simulink library "HDL_ieee_8021513"  (R2024a)
settings: Solver=FixedStepDiscrete  StartTime=0.0  StopTime=10.0  RelTol=1e-3
undefined symbols (not defined in the file or in its folder): Add, axiWidth, channelCyclicPrefixLen, channelDataCarriers, channelEstReference, channelLUT, channelOFDMSamples, channelScramblerInit, decimatorDelay, decimatorFilter, fPHY, frequencyOffsetTimeWindow, fs, headerBitsPerFec, headerBitsPerOFDMSymbol, headerBitsPerSubcarrier, headerCyclicPrefixLen, headerDataCarriers, headerOFDMSamples, headerScramblerInit, interpolatorDelay, interpolatorFilter, leftGuard, N, ncoCarrierFrequency, ncoWordLength, numDataCarriers, oversamplingFactor, payloadBitsPerFec, payloadScramblerInit, payloadWordsPerBlock0, peakDetectorThreshold, peakDetectorWindow, preambleCyclicPrefixLen, preambleDataCarriers, preambleLUT, preambleOFDMSamples, preambleScramblerInit, QAM, rightGuard, Shift
libraries: hdlsllib x198, $bdroot x80, whdlutilities x28, whdledac x10, whdlmod x7, simulink x4, dsphdlfiltering2 x2, dsphdlsigops2 x2, commhdlcrc x2, dspsigops x2, dspstat3 x2, commdigbbndam3 x2
(part 3 of 5)

== system HDL_ieee_8021513/qam_mod ==
  data_in : Inport
  valid_in : Inport  Port=2
  bits_per_subcarrier : Inport  Port=3
  BPSK Modulator Baseband : commdigbbndpm3/BPSK Modulator Baseband  Ph=0  outDtype=Fixed-point  outWordLen=16  outUDDataType=sfix(16)  outFracLenMode=User-defined  outFracLen=14  outDataTypeStr=fixdt(1,16,14)  outLastDataTypeStr=fixdt(1,16,14)
      settings: LibrarySourceBlock=|
      | commhdldigbbndpm/BPSK
      | Modulator
      | Baseband
  Bit Slice : hdlsllib/Logic and Bit Operations/Bit Slice  lidx=0  ridx=0
  Bit Slice1 : hdlsllib/Logic and Bit Operations/Bit Slice  lidx=1  ridx=0
  Bit Slice2 : hdlsllib/Logic and Bit Operations/Bit Slice  lidx=3  ridx=0
  Constant{1..10} (10 alike) : Constant  Value=0  OutDataTypeStr=Inherit: Inherit via back propagation  SampleTime=-1  LockScale=on
  Delay : Delay  DelayLength=1  InitialCondition=0  UseCircularBuffer=on
  Delay1 : Delay  DelayLength=1  InitialCondition=0  UseCircularBuffer=on
  Multiport Switch : MultiPortSwitch  DataPortOrder=Zero-based contiguous  Inputs=8  zeroidx=on  SaturateOnIntegerOverflow=off
  Real-Imag to Complex{1..5} (5 alike) : RealImagToComplex
  batID 1 : commdigbbndam3/Rectangular QAM Modulator Baseband  M=4  InType=Integer  Enc=User-defined  Mapping=qamTwoBits  PowType=Average Power  MinDist=2  AvgPow=1  PeakPow=1  Ph=0  outDtype=Fixed-point  outWordLen=16  outUDDataType=sfix(16)  outFracLenMode=User-defined  outFracLen=14  outDataTypeStr=fixdt(1,16,14)  outLastDataTypeStr=fixdt(1,16,14)
      settings: LibrarySourceBlock=|
      | commhdldigbbndam/Rectangular QAM
      | Modulator
      | Baseband
  batID 8 : commdigbbndam3/Rectangular QAM Modulator Baseband  M=16  InType=Integer  Enc=User-defined  Mapping=qamFourBits  PowType=Average Power  MinDist=2  AvgPow=1  PeakPow=1  Ph=0  outDtype=Fixed-point  outWordLen=16  outUDDataType=sfix(16)  outFracLenMode=User-defined  outFracLen=14  outDataTypeStr=fixdt(1,16,14)  outLastDataTypeStr=fixdt(1,16,14)
      settings: LibrarySourceBlock=|
      | commhdldigbbndam/Rectangular QAM
      | Modulator
      | Baseband
  data_out : Outport
  valid_out : Outport  Port=2  VectorParamsAs1DForOutWhenUnconnected=off
  wires:
  Real-Imag to Complex5/1 -> Multiport Switch/8
  Constant10/1 -> Real-Imag to Complex5/2
  Constant9/1 -> Real-Imag to Complex5/1
  Constant1/1 -> Real-Imag to Complex4/1
  Constant8/1 -> Real-Imag to Complex4/2
  Constant6/1 -> Real-Imag to Complex3/1
  Constant7/1 -> Real-Imag to Complex3/2
  Constant2/1 -> Real-Imag to Complex2/1
  Constant4/1 -> Real-Imag to Complex2/2
  Constant5/1 -> Real-Imag to Complex1/2
  Real-Imag to Complex1/1 -> Multiport Switch/2
  Constant3/1 -> Real-Imag to Complex1/1
  BPSK Modulator Baseband/1 -> Multiport Switch/3
  Delay/1 -> data_out/1
  Real-Imag to Complex2/1 -> Multiport Switch/5
  Real-Imag to Complex4/1 -> Multiport Switch/9
  Real-Imag to Complex3/1 -> Multiport Switch/7
  batID 8/1 -> Multiport Switch/6
  batID 1/1 -> Multiport Switch/4
  Bit Slice2/1 -> batID 8/1
  Bit Slice1/1 -> batID 1/1
  Bit Slice/1 -> BPSK Modulator Baseband/1
  Multiport Switch/1 -> Delay/1
  bits_per_subcarrier/1 -> Multiport Switch/1
  data_in/1 -> Bit Slice2/1, Bit Slice/1, Bit Slice1/1
  Delay1/1 -> valid_out/1
  valid_in/1 -> Delay1/1

== system HDL_ieee_8021513/reduced_ldpc ==
  data_in : Inport
  ctrl_in : Inport  Port=2
  code_rate : Inport  Port=3
  block_size : Inport  Port=4
  Hc_12S-B80 : whdledac/LDPC Encoder  ParityCheckMatrix=Hc_12S  BlockSize=80  SimulateUsing=Code generation
  Terminator : Terminator
  Terminator3 : Terminator
  data_out : Outport
  ctrl_out : Outport  Port=2
  next_frame : Outport  Port=3
  wires:
  ctrl_in/1 -> Hc_12S-B80/2
  Hc_12S-B80/3 -> next_frame/1
  code_rate/1 -> Terminator3/1
  block_size/1 -> Terminator/1
  data_in/1 -> Hc_12S-B80/1
  Hc_12S-B80/1 -> data_out/1
  Hc_12S-B80/2 -> ctrl_out/1

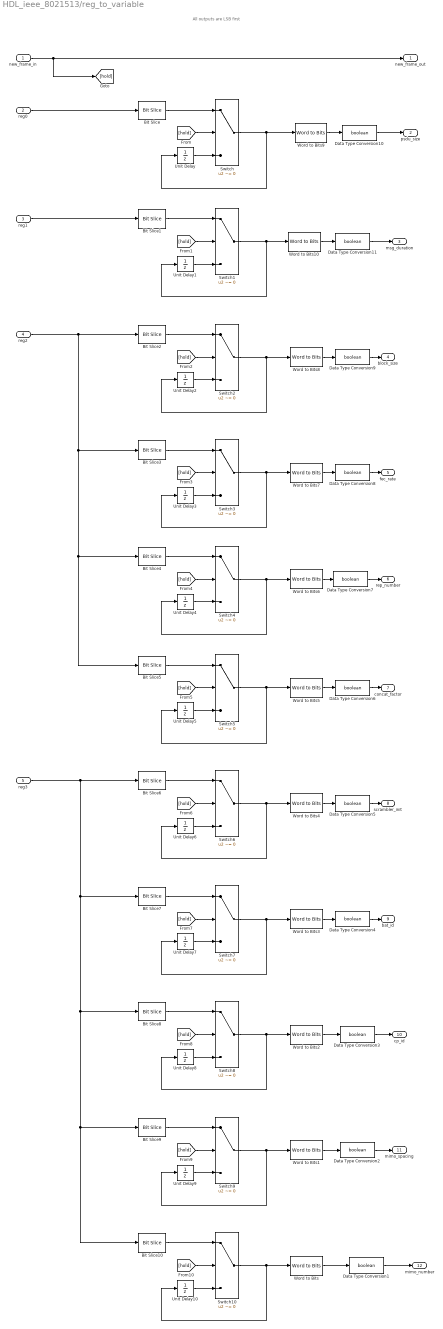
== system HDL_ieee_8021513/reg_to_variable ==
  note: All outputs are LSB first
  new_frame_in : Inport
  reg0 : Inport  Port=2
  reg1 : Inport  Port=3
  reg2 : Inport  Port=4
  reg3 : Inport  Port=5
  Bit Slice : hdlsllib/Logic and Bit Operations/Bit Slice  lidx=23  ridx=0
  Bit Slice1 : hdlsllib/Logic and Bit Operations/Bit Slice  lidx=15  ridx=0
  Bit Slice10 : hdlsllib/Logic and Bit Operations/Bit Slice  lidx=29  ridx=27
  Bit Slice2 : hdlsllib/Logic and Bit Operations/Bit Slice  lidx=1  ridx=0
  Bit Slice3 : hdlsllib/Logic and Bit Operations/Bit Slice  lidx=10  ridx=8
  Bit Slice4 : hdlsllib/Logic and Bit Operations/Bit Slice  lidx=18  ridx=16
  Bit Slice5 : hdlsllib/Logic and Bit Operations/Bit Slice  lidx=26  ridx=24
  Bit Slice6 : hdlsllib/Logic and Bit Operations/Bit Slice  lidx=3  ridx=0
  Bit Slice7 : hdlsllib/Logic and Bit Operations/Bit Slice  lidx=12  ridx=8
  Bit Slice8 : hdlsllib/Logic and Bit Operations/Bit Slice  lidx=18  ridx=16
  Bit Slice9 : hdlsllib/Logic and Bit Operations/Bit Slice  lidx=26  ridx=24
  Data Type Conversion{1..11} (11 alike) : DataTypeConversion  OutDataTypeStr=boolean  SaturateOnIntegerOverflow=off  RndMeth=Floor
  Switch{,1..10} (11 alike) : Switch  Criteria=u2 ~= 0  SaturateOnIntegerOverflow=off  InputSameDT=off
  Unit Delay{,1..10} (11 alike) : UnitDelay  SampleTime=-1  HasFrameUpgradeWarning=on
  Word to Bits{,1..2,5..7} (6 alike) : hdlsllib/Logic and Bit Operations/Word to Bits  maxWordLength=3
  Word to Bits10 : hdlsllib/Logic and Bit Operations/Word to Bits  maxWordLength=16
  Word to Bits3 : hdlsllib/Logic and Bit Operations/Word to Bits  maxWordLength=5
  Word to Bits4 : hdlsllib/Logic and Bit Operations/Word to Bits  maxWordLength=4
  Word to Bits8 : hdlsllib/Logic and Bit Operations/Word to Bits  maxWordLength=2
  Word to Bits9 : hdlsllib/Logic and Bit Operations/Word to Bits  maxWordLength=24
  new_frame_out : Outport  VectorParamsAs1DForOutWhenUnconnected=off
  psdu_size : Outport  Port=2  VectorParamsAs1DForOutWhenUnconnected=off
  msg_duration : Outport  Port=3  VectorParamsAs1DForOutWhenUnconnected=off
  block_size : Outport  Port=4  VectorParamsAs1DForOutWhenUnconnected=off
  fec_rate : Outport  Port=5  VectorParamsAs1DForOutWhenUnconnected=off
  rep_number : Outport  Port=6  VectorParamsAs1DForOutWhenUnconnected=off
  concat_factor : Outport  Port=7  VectorParamsAs1DForOutWhenUnconnected=off
  scrambler_init : Outport  Port=8  VectorParamsAs1DForOutWhenUnconnected=off
  bat_id : Outport  Port=9  VectorParamsAs1DForOutWhenUnconnected=off
  cp_id : Outport  Port=10  VectorParamsAs1DForOutWhenUnconnected=off
  mimo_spacing : Outport  Port=11  VectorParamsAs1DForOutWhenUnconnected=off
  mimo_number : Outport  Port=12  VectorParamsAs1DForOutWhenUnconnected=off
  wires:
  reg3/1 -> Bit Slice10/1, Bit Slice9/1, Bit Slice8/1, Bit Slice7/1, Bit Slice6/1
  reg2/1 -> Bit Slice5/1, Bit Slice4/1, Bit Slice3/1, Bit Slice2/1
  Bit Slice/1 -> Switch/1
  reg1/1 -> Bit Slice1/1
  Unit Delay/1 -> Switch/3
  [hold] -> Switch/2
  reg0/1 -> Bit Slice/1
  Bit Slice1/1 -> Switch1/1
  Unit Delay1/1 -> Switch1/3
  [hold] -> Switch1/2
  [hold] -> Switch2/2
  Unit Delay2/1 -> Switch2/3
  Bit Slice2/1 -> Switch2/1
  Switch2/1 -> Word to Bits8/1, Unit Delay2/1
  Bit Slice3/1 -> Switch3/1
  Switch3/1 -> Word to Bits7/1, Unit Delay3/1
  Unit Delay3/1 -> Switch3/3
  [hold] -> Switch3/2
  Bit Slice6/1 -> Switch6/1
  Bit Slice7/1 -> Switch7/1
  Unit Delay7/1 -> Switch7/3
  Switch5/1 -> Word to Bits5/1, Unit Delay5/1
  Bit Slice5/1 -> Switch5/1
  Switch6/1 -> Word to Bits4/1, Unit Delay6/1
  Unit Delay5/1 -> Switch5/3
  [hold] -> Switch7/2
  Bit Slice4/1 -> Switch4/1
  [hold] -> Switch5/2
  Unit Delay6/1 -> Switch6/3
  Unit Delay4/1 -> Switch4/3
  Switch4/1 -> Word to Bits6/1, Unit Delay4/1
  [hold] -> Switch4/2
  Switch7/1 -> Word to Bits3/1, Unit Delay7/1
  [hold] -> Switch6/2
  Unit Delay9/1 -> Switch9/3
  Bit Slice9/1 -> Switch9/1
  [hold] -> Switch9/2
  [hold] -> Switch8/2
  [hold] -> Switch10/2
  Switch9/1 -> Word to Bits1/1, Unit Delay9/1
  Unit Delay8/1 -> Switch8/3
  Bit Slice8/1 -> Switch8/1
  Bit Slice10/1 -> Switch10/1
  Switch8/1 -> Word to Bits2/1, Unit Delay8/1
  Unit Delay10/1 -> Switch10/3
  Switch10/1 -> Word to Bits/1, Unit Delay10/1
  new_frame_in/1 -> new_frame_out/1, [hold]
  Word to Bits/1 -> Data Type Conversion1/1
  Word to Bits1/1 -> Data Type Conversion2/1
  Word to Bits2/1 -> Data Type Conversion3/1
  Word to Bits3/1 -> Data Type Conversion4/1
  Word to Bits4/1 -> Data Type Conversion5/1
  Word to Bits5/1 -> Data Type Conversion6/1
  Word to Bits6/1 -> Data Type Conversion7/1
  Word to Bits8/1 -> Data Type Conversion9/1
  Word to Bits7/1 -> Data Type Conversion8/1
  Data Type Conversion1/1 -> mimo_number/1
  Data Type Conversion2/1 -> mimo_spacing/1
  Data Type Conversion3/1 -> cp_id/1
  Data Type Conversion4/1 -> bat_id/1
  Data Type Conversion5/1 -> scrambler_init/1
  Data Type Conversion6/1 -> concat_factor/1
  Data Type Conversion7/1 -> rep_number/1
  Data Type Conversion8/1 -> fec_rate/1
  Data Type Conversion9/1 -> block_size/1
  Switch1/1 -> Word to Bits10/1, Unit Delay1/1
  Switch/1 -> Word to Bits9/1, Unit Delay/1
  Word to Bits9/1 -> Data Type Conversion10/1
  Data Type Conversion10/1 -> psdu_size/1
  Word to Bits10/1 -> Data Type Conversion11/1
  Data Type Conversion11/1 -> msg_duration/1

== system HDL_ieee_8021513/remove_tone_mapping ==
  data_in : Inport
  valid_in : Inport  Port=2
  newFrame : Inport  Port=3
  psdu_size : Inport  Port=4
  Bits to Word : hdlsllib/Logic and Bit Operations/Bits to Word
  Data Type Conversion : DataTypeConversion  OutDataTypeStr=fixdt(0,1,0)  SaturateOnIntegerOverflow=off  RndMeth=Floor
  Delay : Delay  DelayLength=1  InitialCondition=0  UseCircularBuffer=on
  HDL Counter : hdlsllib/Sources/HDL Counter  CountType=Free running  CountInit=0  CountStep=1  CountMax=25  CountFromType=Initial value  CountFrom=0  CountResetPort=on  CountLoadPort=off  CountEnbPort=on  CountDirPort=off  CountHitOutputPort=off  CountDataType=Unsigned  CountWordLen=32  CountFracLen=0  CountSampTime=1
  Logical Operator : Logic  IconShape=distinctive  AllPortsSameDT=off  OutDataTypeStr=boolean
  Multiply by 2 (for fec_rate 1/2) : hdlsllib/Logic and Bit Operations/Bit Shift  mode=Shift Left Logical  N=1
  Multiply by 8 : hdlsllib/Logic and Bit Operations/Bit Shift  mode=Shift Left Logical  N=3
  Relational Operator : RelationalOperator  Operator=<  OutDataTypeStr=boolean  InputSameDT=off
  valid_to_ctrl : $bdroot/valid_to_ctrl  SystemSampleTime=-1  VariantActivationTime=update diagram  AllowFlexibleInterface=on  Latency=0  AutoFrameSizeCalculation=off
  data_out : Outport
  ctrl_out : Outport  Port=2
  wires:
  newFrame/1 -> HDL Counter/1
  Multiply by 2 (for fec_rate 1/2)/1 -> Relational Operator/2
  Delay/1 -> data_out/1
  valid_to_ctrl/1 -> ctrl_out/1
  psdu_size/1 -> Data Type Conversion/1
  Bits to Word/1 -> Multiply by 8/1
  HDL Counter/1 -> Relational Operator/1  "Count"
  Multiply by 8/1 -> Multiply by 2 (for fec_rate 1/2)/1
  Logical Operator/1 -> valid_to_ctrl/1  "valid_out"
  Relational Operator/1 -> Logical Operator/2
  Data Type Conversion/1 -> Bits to Word/1
  valid_in/1 -> HDL Counter/2, Logical Operator/1
  data_in/1 -> Delay/1

== system HDL_ieee_8021513/rising_edge_detector ==
  In : Inport
  Delay2 : Delay  DelayLength=1  InitialCondition=0  UseCircularBuffer=on
  Logical Operator1 : Logic  IconShape=distinctive  AllPortsSameDT=off  OutDataTypeStr=boolean
  Logical Operator2 : Logic  Operator=NOT  IconShape=distinctive  AllPortsSameDT=off  OutDataTypeStr=boolean
  Out : Outport
  wires:
  Logical Operator2/1 -> Logical Operator1/2
  Delay2/1 -> Logical Operator2/1
  In/1 -> Logical Operator1/1, Delay2/1
  Logical Operator1/1 -> Out/1

== system HDL_ieee_8021513/rx_demodulator_full ==
  note: Last frame has one less delay because of the falling edge
  data_in : Inport
  payload_cp_len : Inport  Port=2
  payload_bits_per_subcarrier : Inport  Port=3
  psdu_size : Inport  Port=4
  header_ready : Inport  Port=5
  AND1 : Logic  IconShape=distinctive  AllPortsSameDT=off  OutDataTypeStr=boolean
  AND2 : Logic  IconShape=distinctive  AllPortsSameDT=off  OutDataTypeStr=boolean
  Constant : Constant  Value=0  OutDataTypeStr=boolean  SampleTime=-1
  Constant1 : Constant  OutDataTypeStr=boolean  SampleTime=-1
  Delay : Delay  DelayLength=1  InitialCondition=0  UseCircularBuffer=on
  Delay1 : Delay  DelayLength=3  InitialCondition=0  UseCircularBuffer=on
  Delay15 : Delay  DelayLength=3  InitialCondition=0  UseCircularBuffer=on
  Delay16 : Delay  InitialCondition=0  UseCircularBuffer=on
  Delay17 : Delay  DelayLength=100  InitialCondition=0  UseCircularBuffer=on
  Delay18 : Delay  DelayLength=7  InitialCondition=0  UseCircularBuffer=on
  Delay19 : Delay  DelayLength=7  InitialCondition=0  UseCircularBuffer=on
  Delay20 : Delay  DelayLength=7  InitialCondition=0  UseCircularBuffer=on
  Delay4 : Delay  DelayLength=100  InitialCondition=0  UseCircularBuffer=on
  Delay5 : Delay  DelayLength=1  InitialCondition=0  UseCircularBuffer=on
  Delay6 : Delay  DelayLength=1  InitialCondition=0  UseCircularBuffer=on
  Delay7 : Delay  DelayLength=100  InitialCondition=0  UseCircularBuffer=on
  Delay8 : Delay  DelayLength=3  InitialCondition=0  UseCircularBuffer=on
  Logical Operator : Logic  IconShape=distinctive  AllPortsSameDT=off  OutDataTypeStr=boolean
  Logical Operator1 : Logic  Operator=OR  Inputs=3  IconShape=distinctive  AllPortsSameDT=off  OutDataTypeStr=boolean
  Logical Operator6 : Logic  IconShape=distinctive  AllPortsSameDT=off  OutDataTypeStr=boolean
  Logical Operator7 : Logic  IconShape=distinctive  AllPortsSameDT=off  OutDataTypeStr=boolean
  OR : Logic  Operator=OR  IconShape=distinctive  AllPortsSameDT=off  OutDataTypeStr=boolean
  Rate Transition : RateTransition  OutPortSampleTime=1/fs
  Terminator : Terminator
  Terminator1 : Terminator
  Terminator2 : Terminator
  channel_estimation_and_equalization : $bdroot/channel_estimation_and_equalization  SystemSampleTime=-1  VariantActivationTime=update diagram  AllowFlexibleInterface=on  Latency=0  AutoFrameSizeCalculation=off
  constellation_descrambler : $bdroot/constellation_descrambler  SystemSampleTime=-1  VariantActivationTime=update diagram  AllowFlexibleInterface=on  Latency=0  AutoFrameSizeCalculation=off
  decimator : $bdroot/decimator  SystemSampleTime=-1  VariantActivationTime=update diagram  AllowFlexibleInterface=on  Latency=0  AutoFrameSizeCalculation=off
  downshifter : $bdroot/downshifter  SystemSampleTime=-1  VariantActivationTime=update diagram  AllowFlexibleInterface=on  Latency=0  AutoFrameSizeCalculation=off
  get_bits_per_subcarrier : Subsystem
  get_cp : Subsystem
  get_init : Subsystem
  ofdm_demod : $bdroot/ofdm_demod  SystemSampleTime=-1  VariantActivationTime=update diagram  AllowFlexibleInterface=on  Latency=0  AutoFrameSizeCalculation=off
  ofdm_rx_counter : Subsystem
  ofdm_separator : $bdroot/ofdm_separator  SystemSampleTime=-1  VariantActivationTime=update diagram  AllowFlexibleInterface=on  Latency=0  AutoFrameSizeCalculation=off
  ofdm_symbol_sync : $bdroot/ofdm_symbol_sync  SystemSampleTime=-1  VariantActivationTime=update diagram  AllowFlexibleInterface=on  Latency=0  AutoFrameSizeCalculation=off
  qam_demod : $bdroot/qam_demod  SystemSampleTime=-1  VariantActivationTime=update diagram  AllowFlexibleInterface=on  Latency=0  AutoFrameSizeCalculation=off
  data_out : Outport  VectorParamsAs1DForOutWhenUnconnected=off
  valid_header : Outport  Port=2  VectorParamsAs1DForOutWhenUnconnected=off
  valid_payload : Outport  Port=3  VectorParamsAs1DForOutWhenUnconnected=off
  last_frame : Outport  Port=4  VectorParamsAs1DForOutWhenUnconnected=off
  wires:
  [reset] -> channel_estimation_and_equalization/5
  [reset] -> ofdm_demod/4
  ofdm_symbol_sync/5 -> [reset]
  header_ready/1 -> ofdm_separator/6
  ofdm_separator/4 -> get_cp/2(valid_payload), Logical Operator1/3  "valid_payload"
  Delay17/1 -> Delay20/1
  Delay7/1 -> Delay19/1
  Delay4/1 -> get_bits_per_subcarrier/2(valid_header), Delay18/1
  Delay16/1 -> Delay17/1
  Delay1/1 -> AND1/2
  ofdm_symbol_sync/3 -> [freq_offset]
  ofdm_symbol_sync/4 -> Terminator1/1
  [p_bits] -> get_bits_per_subcarrier/1(payload_bits_per_sub)
  [p_cp] -> get_cp/3(cp_payload)
  channel_estimation_and_equalization/1 -> qam_demod/1
  channel_estimation_and_equalization/2 -> qam_demod/2
  channel_estimation_and_equalization/3 -> Terminator/1
  Constant/1 -> channel_estimation_and_equalization/4
  constellation_descrambler/1 -> channel_estimation_and_equalization/1
  AND2/1 -> channel_estimation_and_equalization/2
  AND1/1 -> channel_estimation_and_equalization/3
  OR/1 -> AND2/1
  Delay15/1 -> Delay7/1, OR/2
  Delay8/1 -> Delay4/1, OR/1
  ofdm_rx_counter/1(is_channel) -> Delay1/1  "is_channel"
  get_bits_per_subcarrier/1(qam_demod_bits) -> qam_demod/3
  ofdm_rx_counter/3(is_payload) -> Delay15/1, get_init/2(valid_payload)  "is_payload"
  ofdm_rx_counter/2(is_header) -> Delay8/1, get_init/1(valid_header)  "is_header"
  get_init/1(descrambler_init) -> constellation_descrambler/3
  get_cp/1(ofdm_cp_len) -> ofdm_demod/3  "cp_len"
  ofdm_separator/5 -> ofdm_rx_counter/3(payload_num_ofdm_symbols)
  ofdm_separator/3 -> get_cp/1(valid_header), Logical Operator1/2  "valid_header"
  ofdm_separator/2 -> Logical Operator1/1, ofdm_rx_counter/2(rst)  "valid_channel"
  ofdm_symbol_sync/1 -> ofdm_separator/1
  ofdm_symbol_sync/2 -> ofdm_separator/2  "peak_sync"
  ofdm_separator/1 -> ofdm_demod/1
  decimator/1 -> ofdm_symbol_sync/1
  Delay19/1 -> Logical Operator7/2
  Delay18/1 -> Logical Operator6/2
  ofdm_rx_counter/4(last_frame) -> Delay16/1  "last_frame"
  qam_demod/2 -> Logical Operator7/1, Logical Operator6/1
  Logical Operator6/1 -> valid_header/1
  Logical Operator7/1 -> valid_payload/1
  Delay20/1 -> last_frame/1
  ofdm_demod/3 -> Delay/1
  constellation_descrambler/2 -> AND1/1, AND2/2  "qam_demod_valid"
  data_in/1 -> downshifter/1
  Logical Operator/1 -> ofdm_demod/2  "ofdm_valid"
  ofdm_demod/2 -> ofdm_rx_counter/1(valid), Delay5/1  "valid_ofdm_demod_out"
  Delay/1 -> Logical Operator/1
  ofdm_demod/1 -> Delay6/1
  psdu_size/1 -> ofdm_separator/3
  payload_bits_per_subcarrier/1 -> [p_bits], ofdm_separator/4
  payload_cp_len/1 -> ofdm_separator/5, [p_cp]
  Logical Operator1/1 -> Logical Operator/2
  downshifter/1 -> decimator/1
  downshifter/2 -> decimator/2
  Delay5/1 -> constellation_descrambler/2  "descrambler_valid"
  Delay6/1 -> constellation_descrambler/1
  qam_demod/1 -> data_out/1
  [freq_offset] -> Rate Transition/1
  Constant1/1 -> downshifter/2
  Rate Transition/1 -> downshifter/3
  decimator/2 -> Terminator2/1

== system HDL_ieee_8021513/rx_payload_full ==
  note: Note: this blocks requires exactly one external delay for signals "data_in" and "valid_in"
  data_in : Inport
  valid_in : Inport  Port=2
  last_frame : Inport  Port=3
  new_frame : Inport  Port=4
  scrambler_init : Inport  Port=5
  fec_rate : Inport  Port=6
  block_size : Inport  Port=7
  psdu_size : Inport  Port=8
  AND : Logic  IconShape=distinctive  AllPortsSameDT=off  OutDataTypeStr=boolean
  Bits to Word : hdlsllib/Logic and Bit Operations/Bits to Word
  Data Type Conversion : DataTypeConversion  OutDataTypeStr=uint8  SaturateOnIntegerOverflow=off  RndMeth=Floor
  Data Type Conversion1 : DataTypeConversion  OutDataTypeStr=fixdt(0,1,0)  SaturateOnIntegerOverflow=off  RndMeth=Floor
  Delay : Delay  DelayLength=1  InitialCondition=0  UseCircularBuffer=on
  Delay3 : Delay  DelayLength=1  InitialCondition=0  UseCircularBuffer=on
  Delay4 : Delay  DelayLength=1  InitialCondition=0  UseCircularBuffer=on
  Deserializer1D : hdlsllib/HDL Operations/Deserializer1D  Ratio=8  IdleCycles=0  InitialCondition=0  startIn=off  validIn=on  validOut=on  inputDataDimensions=-1  inputSampleTime=-1  inputSignalType=auto
  Logical Operator1 : Logic  IconShape=distinctive  AllPortsSameDT=off  OutDataTypeStr=boolean
  Logical Operator5 : Logic  Operator=OR  IconShape=distinctive  AllPortsSameDT=off  OutDataTypeStr=boolean
  Sample Control Bus Selector : whdlutilities/Sample Control Bus Selector  OutputSignals=start,end,valid
  Switch1 : Switch  Criteria=u2 ~= 0  SaturateOnIntegerOverflow=off  InputSameDT=off
  Terminator : Terminator
  Terminator1 : Terminator
  Unit Delay1 : UnitDelay  SampleTime=-1  HasFrameUpgradeWarning=on
  next_frame_to_ready_rx : Subsystem
  p_scrambler : $bdroot/p_scrambler  SystemSampleTime=-1  VariantActivationTime=update diagram  AllowFlexibleInterface=on  Latency=0  AutoFrameSizeCalculation=off
      settings: LibrarySourceBlock=|
      | hdlsllib/Ports &
      | Subsystems/Subsystem
  reduced_ldpc_rx : Subsystem
  remove_tone_mapping : $bdroot/remove_tone_mapping  SystemSampleTime=-1  VariantActivationTime=update diagram  AllowFlexibleInterface=on  Latency=0  AutoFrameSizeCalculation=off
  data_out : Outport  VectorParamsAs1DForOutWhenUnconnected=off
  valid_out : Outport  Port=2  VectorParamsAs1DForOutWhenUnconnected=off
  ready : Outport  Port=3  VectorParamsAs1DForOutWhenUnconnected=off
  wires:
  p_scrambler/2 -> Sample Control Bus Selector/1
  Sample Control Bus Selector/2 -> Terminator/1
  Sample Control Bus Selector/1 -> Terminator1/1
  block_size/1 -> reduced_ldpc_rx/4(block_size)
  fec_rate/1 -> reduced_ldpc_rx/3(fec_rate)
  scrambler_init/1 -> p_scrambler/3
  reduced_ldpc_rx/2(ctrl_out) -> p_scrambler/2  "ldpc_ctrl_out"
  reduced_ldpc_rx/1(data_out) -> p_scrambler/1  "ldpc_out"
  psdu_size/1 -> remove_tone_mapping/4
  remove_tone_mapping/1 -> reduced_ldpc_rx/1(data_in)  "ldpc_in"
  remove_tone_mapping/2 -> reduced_ldpc_rx/2(ctrl_in)  "ldpc_ctrl_in"
  reduced_ldpc_rx/3(next_frame) -> Delay/1
  next_frame_to_ready_rx/1(ready) -> Delay3/1, ready/1  "ready"
  data_in/1 -> remove_tone_mapping/1
  AND/1 -> remove_tone_mapping/2
  valid_in/1 -> AND/2
  Delay3/1 -> AND/1
  Logical Operator5/1 -> Switch1/2
  new_frame/1 -> [new_frame], Switch1/1, Logical Operator5/1
  Unit Delay1/1 -> Switch1/3
  last_frame/1 -> Delay4/1
  Logical Operator1/1 -> next_frame_to_ready_rx/1(next_frame)
  Switch1/1 -> Logical Operator1/1, Unit Delay1/1
  Delay/1 -> Logical Operator1/2
  Delay4/1 -> Logical Operator5/2
  [new_frame] -> remove_tone_mapping/3
  Deserializer1D/1 -> Data Type Conversion1/1
  Sample Control Bus Selector/3 -> Deserializer1D/2
  Data Type Conversion/1 -> data_out/1
  Deserializer1D/2 -> valid_out/1
  p_scrambler/1 -> Deserializer1D/1
  Bits to Word/1 -> Data Type Conversion/1
  Data Type Conversion1/1 -> Bits to Word/1

== system HDL_ieee_8021513/sync_constellation_scrambler ==
  new_ofdm_symbol : Inport
  init : Inport  Port=2
  valid_in : Inport  Port=3
  Rate Transition : RateTransition  OutPortSampleTime=1/fPHY
  Rate Transition1 : RateTransition  OutPortSampleTime=1/fPHY
  Rate Transition2 : RateTransition  OutPortSampleTime=1/(2*fPHY)
  Rate Transition3 : RateTransition  OutPortSampleTime=1/(2*fPHY)
  Rate Transition4 : RateTransition  OutPortSampleTime=1/(2*fPHY)
  Synchronous constellation scrambler : Subsystem
  s1 : Outport  VectorParamsAs1DForOutWhenUnconnected=off
  s2 : Outport  Port=2  VectorParamsAs1DForOutWhenUnconnected=off
  wires:
  Rate Transition4/1 -> Synchronous constellation scrambler/1(valid_in)
  Rate Transition3/1 -> Synchronous constellation scrambler/2(init)
  Synchronous constellation scrambler/1(s1_out) -> Rate Transition1/1
  Synchronous constellation scrambler/2(s2_out) -> Rate Transition/1
  Rate Transition2/1 -> Synchronous constellation scrambler/3(new_ofdm_symbol)
  new_ofdm_symbol/1 -> Rate Transition2/1
  valid_in/1 -> Rate Transition4/1
  init/1 -> Rate Transition3/1
  Rate Transition1/1 -> s1/1
  Rate Transition/1 -> s2/1

== system HDL_ieee_8021513/tone_mapping ==
  data_in : Inport
  ctrl_in : Inport  Port=2
  bits_per_subcarrier : Inport  Port=3
  len_in_ofdm_symbols : Inport  Port=4
  new_frame : Inport  Port=5
  Compare To Constant : hdlsllib/Logic and Bit Operations/Compare To Constant  relop===  const=1  OutDataTypeStr=boolean
  Constant : Constant  Value=0  OutDataTypeStr=boolean  SampleTime=-1
  Data Type Conversion : DataTypeConversion  OutDataTypeStr=uint8  SaturateOnIntegerOverflow=off  RndMeth=Floor
  Delay{,1..10} (11 alike) : Delay  DelayLength=1  InitialCondition=0  UseCircularBuffer=on
  Gain : Gain  Gain=numDataCarriers  OutDataTypeStr=fixdt(0,10,0)
  HDL Counter : hdlsllib/Sources/HDL Counter  CountType=Free running  CountInit=0  CountStep=1  CountMax=numDataCarriers-1  CountFromType=Initial value  CountFrom=0  CountResetPort=on  CountLoadPort=off  CountEnbPort=on  CountDirPort=off  CountHitOutputPort=off  CountDataType=Unsigned  CountWordLen=32  CountFracLen=0  CountSampTime=1
  Logical Operator : Logic  AllPortsSameDT=off  OutDataTypeStr=boolean
  Logical Operator1 : Logic  IconShape=distinctive  AllPortsSameDT=off  OutDataTypeStr=boolean
  Logical Operator{2,4,6..7} (4 alike) : Logic  Operator=OR  IconShape=distinctive  AllPortsSameDT=off  OutDataTypeStr=boolean
  Logical Operator3 : Logic  IconShape=distinctive  AllPortsSameDT=off  OutDataTypeStr=boolean
  Logical Operator5 : Logic  IconShape=distinctive  AllPortsSameDT=off  OutDataTypeStr=boolean
  Product1 : Product
  Relational Operator : RelationalOperator  Operator=<=  OutDataTypeStr=boolean  InputSameDT=off
  Sample Control Bus Creator : whdlutilities/Sample Control Bus Creator
  Sample Control Bus Selector : whdlutilities/Sample Control Bus Selector  OutputSignals=start,end,valid
  Subtract : Sum  Inputs=+-  OutDataTypeStr=Inherit: Same as first input
  Switch : Switch  Criteria=u2 ~= 0  SaturateOnIntegerOverflow=off  InputSameDT=off
  Switch1 : Switch  Criteria=u2 ~= 0  SaturateOnIntegerOverflow=off  InputSameDT=off
  Switch2 : Switch  Criteria=u2 ~= 0  SaturateOnIntegerOverflow=off  InputSameDT=off
  Unit Delay1 : UnitDelay  SampleTime=-1  HasFrameUpgradeWarning=on
  Unit Delay2 : UnitDelay  SampleTime=-1  HasFrameUpgradeWarning=on
  data_out : Outport
  ctrl_out : Outport  Port=2
  wires:
  Data Type Conversion/1 -> Gain/1
  Delay2/1 -> Logical Operator7/1
  Logical Operator1/1 -> Delay3/1
  Logical Operator7/1 -> Switch1/2
  Sample Control Bus Selector/1 -> Logical Operator1/2, Delay2/1
  Unit Delay2/1 -> Switch1/3
  Switch1/1 -> Unit Delay2/1, Logical Operator1/1  "new_frame_hold"
  Sample Control Bus Selector/2 -> Logical Operator/1
  Relational Operator/1 -> Logical Operator/2
  Logical Operator/1 -> Switch2/1, Logical Operator6/2
  new_frame/1 -> Logical Operator7/2, Switch1/1, HDL Counter/1  "new_frame"
  Switch/1 -> data_out/1
  ctrl_in/1 -> Delay7/1
  Sample Control Bus Selector/3 -> Delay10/1
  Sample Control Bus Creator/1 -> ctrl_out/1
  Logical Operator2/1 -> Sample Control Bus Creator/3
  Unit Delay1/1 -> Switch2/3
  Switch2/1 -> Delay1/1, Unit Delay1/1
  Logical Operator3/1 -> Sample Control Bus Creator/2
  Logical Operator4/1 -> HDL Counter/2  "enable"
  [hold_end] -> Logical Operator4/2
  Constant/1 -> Switch/1
  data_in/1 -> Delay6/1
  [hold_end] -> Logical Operator3/2
  HDL Counter/1 -> Subtract/2  "count"
  Delay/1 -> Switch/3
  Delay1/1 -> [hold_end], Logical Operator5/2, Logical Operator2/2  "hold_end"
  Delay10/1 -> Logical Operator4/1, Logical Operator2/1
  Delay3/1 -> Sample Control Bus Creator/1
  Logical Operator6/1 -> Switch2/2
  Logical Operator5/1 -> Logical Operator6/1
  [hold_end] -> Delay4/1
  Delay4/1 -> Switch/2
  Subtract/1 -> Relational Operator/1, Compare To Constant/1
  Compare To Constant/1 -> Logical Operator5/1, Logical Operator3/1
  bits_per_subcarrier/1 -> Data Type Conversion/1
  Delay5/1 -> [count_hit]  "count_hit"
  [count_hit] -> Subtract/1
  Delay6/1 -> Delay/1
  Delay7/1 -> Sample Control Bus Selector/1
  Gain/1 -> Delay8/1
  Delay8/1 -> Product1/1, Relational Operator/2
  len_in_ofdm_symbols/1 -> Delay9/1
  Product1/1 -> Delay5/1
  Delay9/1 -> Product1/2

== system HDL_ieee_8021513/valid_to_ctrl ==
  validIn : Inport
  Delay1 : Delay  DelayLength=1  InitialCondition=0  UseCircularBuffer=on
  Delay2 : Delay  DelayLength=1  InitialCondition=0  UseCircularBuffer=on
  Logical Operator : Logic  IconShape=distinctive  AllPortsSameDT=off  OutDataTypeStr=boolean
  Logical Operator1 : Logic  Operator=NOT  IconShape=distinctive  AllPortsSameDT=off  OutDataTypeStr=boolean
  Logical Operator2 : Logic  IconShape=distinctive  AllPortsSameDT=off  OutDataTypeStr=boolean
  Logical Operator3 : Logic  Operator=NOT  IconShape=distinctive  AllPortsSameDT=off  OutDataTypeStr=boolean
  Sample Control Bus Creator : whdlutilities/Sample Control Bus Creator
  ctrlOut : Outport  VectorParamsAs1DForOutWhenUnconnected=off
  wires:
  validIn/1 -> Logical Operator3/1, Delay1/1
  Logical Operator3/1 -> Logical Operator2/2
  Delay2/1 -> Logical Operator1/1
  Logical Operator1/1 -> Logical Operator/2
  Delay1/1 -> Logical Operator/1, Sample Control Bus Creator/3, Logical Operator2/1, Delay2/1  "valid"
  Logical Operator/1 -> Sample Control Bus Creator/1  "start"
  Logical Operator2/1 -> Sample Control Bus Creator/2  "end"
  Sample Control Bus Creator/1 -> ctrlOut/1

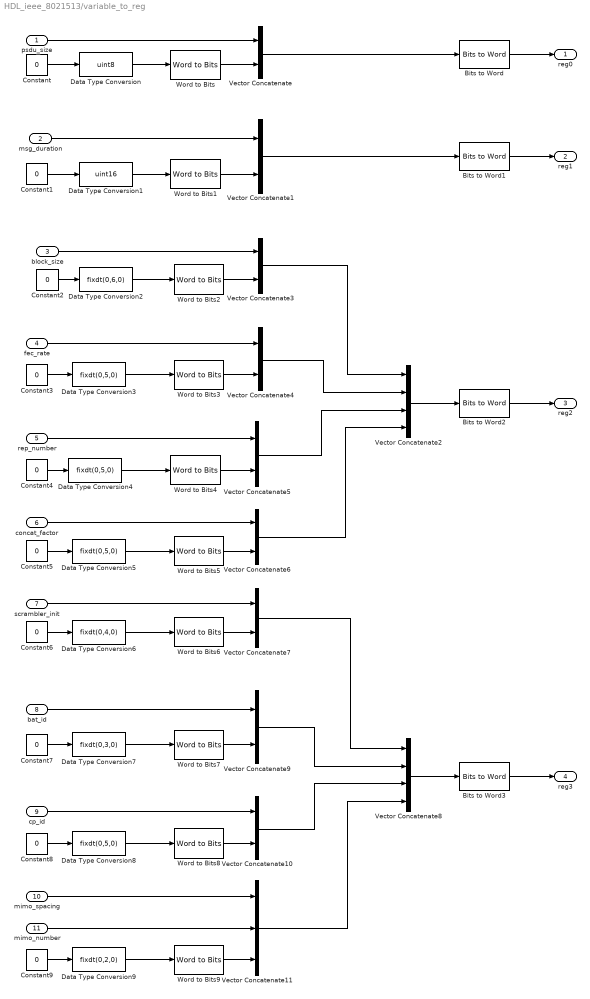
== system HDL_ieee_8021513/variable_to_reg ==
  psdu_size : Inport
  msg_duration : Inport  Port=2
  block_size : Inport  Port=3
  fec_rate : Inport  Port=4
  rep_number : Inport  Port=5
  concat_factor : Inport  Port=6
  scrambler_init : Inport  Port=7
  bat_id : Inport  Port=8
  cp_id : Inport  Port=9
  mimo_spacing : Inport  Port=10
  mimo_number : Inport  Port=11
  Bits to Word{,1..3} (4 alike) : hdlsllib/Logic and Bit Operations/Bits to Word
  Constant : Constant  Value=0  OutDataTypeStr=uint8  SampleTime=-1
  Constant1 : Constant  Value=0  OutDataTypeStr=uint16  SampleTime=-1
  Constant2 : Constant  Value=0  OutDataTypeStr=fixdt(0,6,0)  SampleTime=-1
  Constant{3..5,8} (4 alike) : Constant  Value=0  OutDataTypeStr=fixdt(0,5,0)  SampleTime=-1
  Constant6 : Constant  Value=0  OutDataTypeStr=fixdt(0,4,0)  SampleTime=-1
  Constant7 : Constant  Value=0  OutDataTypeStr=fixdt(0,3,0)  SampleTime=-1
  Constant9 : Constant  Value=0  OutDataTypeStr=fixdt(0,2,0)  SampleTime=-1
  Data Type Conversion : DataTypeConversion  OutDataTypeStr=uint8  SaturateOnIntegerOverflow=off  RndMeth=Floor
  Data Type Conversion1 : DataTypeConversion  OutDataTypeStr=uint16  SaturateOnIntegerOverflow=off  RndMeth=Floor
  Data Type Conversion2 : DataTypeConversion  OutDataTypeStr=fixdt(0,6,0)  SaturateOnIntegerOverflow=off  RndMeth=Floor
  Data Type Conversion{3..5,8} (4 alike) : DataTypeConversion  OutDataTypeStr=fixdt(0,5,0)  SaturateOnIntegerOverflow=off  RndMeth=Floor
  Data Type Conversion6 : DataTypeConversion  OutDataTypeStr=fixdt(0,4,0)  SaturateOnIntegerOverflow=off  RndMeth=Floor
  Data Type Conversion7 : DataTypeConversion  OutDataTypeStr=fixdt(0,3,0)  SaturateOnIntegerOverflow=off  RndMeth=Floor
  Data Type Conversion9 : DataTypeConversion  OutDataTypeStr=fixdt(0,2,0)  SaturateOnIntegerOverflow=off  RndMeth=Floor
  Vector Concatenate{,1,3..7,9..10} (9 alike) : Concatenate
  Vector Concatenate11 : Concatenate  NumInputs=3
  Vector Concatenate2 : Concatenate  NumInputs=4
  Vector Concatenate8 : Concatenate  NumInputs=4
  Word to Bits : hdlsllib/Logic and Bit Operations/Word to Bits  maxWordLength=8
  Word to Bits1 : hdlsllib/Logic and Bit Operations/Word to Bits  maxWordLength=16
  Word to Bits2 : hdlsllib/Logic and Bit Operations/Word to Bits  maxWordLength=6
  Word to Bits{3..5,8} (4 alike) : hdlsllib/Logic and Bit Operations/Word to Bits  maxWordLength=5
  Word to Bits6 : hdlsllib/Logic and Bit Operations/Word to Bits  maxWordLength=4
  Word to Bits7 : hdlsllib/Logic and Bit Operations/Word to Bits  maxWordLength=3
  Word to Bits9 : hdlsllib/Logic and Bit Operations/Word to Bits  maxWordLength=2
  reg0 : Outport
  reg1 : Outport  Port=2
  reg2 : Outport  Port=3
  reg3 : Outport  Port=4
  wires:
  psdu_size/1 -> Vector Concatenate/1
  Constant/1 -> Data Type Conversion/1
  Word to Bits/1 -> Vector Concatenate/2
  Vector Concatenate/1 -> Bits to Word/1
  Bits to Word/1 -> reg0/1
  Data Type Conversion/1 -> Word to Bits/1
  Constant1/1 -> Data Type Conversion1/1
  Data Type Conversion1/1 -> Word to Bits1/1
  msg_duration/1 -> Vector Concatenate1/1
  Word to Bits1/1 -> Vector Concatenate1/2
  Vector Concatenate1/1 -> Bits to Word1/1
  Bits to Word1/1 -> reg1/1
  Constant2/1 -> Data Type Conversion2/1
  Data Type Conversion2/1 -> Word to Bits2/1
  block_size/1 -> Vector Concatenate3/1
  Word to Bits2/1 -> Vector Concatenate3/2
  Constant3/1 -> Data Type Conversion3/1
  Data Type Conversion3/1 -> Word to Bits3/1
  fec_rate/1 -> Vector Concatenate4/1
  Word to Bits3/1 -> Vector Concatenate4/2
  Vector Concatenate3/1 -> Vector Concatenate2/1
  Vector Concatenate4/1 -> Vector Concatenate2/2
  Vector Concatenate2/1 -> Bits to Word2/1
  Constant4/1 -> Data Type Conversion4/1
  Data Type Conversion4/1 -> Word to Bits4/1
  rep_number/1 -> Vector Concatenate5/1
  Word to Bits4/1 -> Vector Concatenate5/2
  Vector Concatenate5/1 -> Vector Concatenate2/3
  Data Type Conversion5/1 -> Word to Bits5/1
  Constant5/1 -> Data Type Conversion5/1
  concat_factor/1 -> Vector Concatenate6/1
  Word to Bits5/1 -> Vector Concatenate6/2
  Vector Concatenate6/1 -> Vector Concatenate2/4
  Data Type Conversion6/1 -> Word to Bits6/1
  Constant6/1 -> Data Type Conversion6/1
  scrambler_init/1 -> Vector Concatenate7/1
  Word to Bits6/1 -> Vector Concatenate7/2
  Vector Concatenate7/1 -> Vector Concatenate8/1
  Constant7/1 -> Data Type Conversion7/1
  Data Type Conversion7/1 -> Word to Bits7/1
  bat_id/1 -> Vector Concatenate9/1
  Word to Bits7/1 -> Vector Concatenate9/2
  Vector Concatenate9/1 -> Vector Concatenate8/2
  Data Type Conversion8/1 -> Word to Bits8/1
  Constant8/1 -> Data Type Conversion8/1
  cp_id/1 -> Vector Concatenate10/1
  Word to Bits8/1 -> Vector Concatenate10/2
  mimo_spacing/1 -> Vector Concatenate11/1
  mimo_number/1 -> Vector Concatenate11/2
  Constant9/1 -> Data Type Conversion9/1
  Data Type Conversion9/1 -> Word to Bits9/1
  Word to Bits9/1 -> Vector Concatenate11/3
  Vector Concatenate10/1 -> Vector Concatenate8/3
  Vector Concatenate11/1 -> Vector Concatenate8/4
  Vector Concatenate8/1 -> Bits to Word3/1
  Bits to Word2/1 -> reg2/1
  Bits to Word3/1 -> reg3/1

== system HDL_ieee_8021513/calculate_mean_and_std/calculate_mean_x ==
  note: Return:
      | $\sum_{i=0}^{N-1}{x(i)}$
  data_in : Inport
  Add1 : Sum  OutDataTypeStr=Inherit: Same as first input
  Delay : Delay  DelayLength=1  InitialCondition=0  UseCircularBuffer=on
  Delay1 : Delay  DelayLength=1  InitialCondition=0  UseCircularBuffer=on
  Delay2 : Delay  DelayLength=1  InitialCondition=0  UseCircularBuffer=on
  Divide by 1024 : hdlsllib/Logic and Bit Operations/Bit Shift  mode=Shift Right Arithmetic  N=10
  N delay : Delay  DelayLength=1024  InitialCondition=0  UseCircularBuffer=on
  Subtract : Sum  Inputs=+-  OutDataTypeStr=fixdt(1,32,12)
  mean : Outport
  wires:
  data_in/1 -> Delay2/1  "x(i+N)"
  Delay1/1 -> Divide by 1024/1, Add1/2
  N delay/1 -> Subtract/2  "x(i)"
  Add1/1 -> Delay1/1
  Subtract/1 -> Delay/1
  Divide by 1024/1 -> mean/1
  Delay/1 -> Add1/1
  Delay2/1 -> Subtract/1, N delay/1

== system HDL_ieee_8021513/calculate_mean_and_std/calculate_mean_x_squared ==
  note: Return:
      | $\sum_{i=0}^{N-1}{(x(i)^2)}$
  data_in : Inport
  Add1 : Sum  OutDataTypeStr=Inherit: Same as first input
  Delay : Delay  DelayLength=1  InitialCondition=0  UseCircularBuffer=on
  Delay1 : Delay  DelayLength=1  InitialCondition=0  UseCircularBuffer=on
  Delay2 : Delay  DelayLength=1  InitialCondition=0  UseCircularBuffer=on
  Divide by 1024 : hdlsllib/Logic and Bit Operations/Bit Shift  mode=Shift Right Arithmetic  N=10
  N delay : Delay  DelayLength=1024  InitialCondition=0  UseCircularBuffer=on
  Square : Math  Operator=square  SignedPower=on  RndMeth=Zero  OutDataTypeStr=Inherit: Inherit via internal rule
  Subtract : Sum  Inputs=+-
  mean_x_squared : Outport
  wires:
  data_in/1 -> Square/1  "x(i+N)"
  Delay1/1 -> Divide by 1024/1, Add1/2
  N delay/1 -> Subtract/2  "x(i)"
  Add1/1 -> Delay1/1
  Subtract/1 -> Delay/1
  Divide by 1024/1 -> mean_x_squared/1
  Delay/1 -> Add1/1
  Square/1 -> Delay2/1
  Delay2/1 -> Subtract/1, N delay/1

== system HDL_ieee_8021513/channel_estimation_and_equalization/Channel Equalization ==
  data_in : Inport
  valid_data : Inport  Port=2
  channel_estimate_in : Inport  Port=3
  valid_channel_estimate : Inport  Port=4
  dont_use_equalizer : Inport  Port=5
  reset : Inport  Port=6
  Channel Estimates Store RAM : hdlsllib/HDL RAMs/Simple Dual Port RAM System  RAMType=Simple dual port  AsyncRead=off  WriteOutputValue=New data  RAMInitialValue=0  allowBusInputs=off  WritesHaveOutput=on  NumReads=0  NumWrites=1  SimulateUsing=Code generation
  Constant : Constant  Value=numDataCarriers  OutDataTypeStr=fixdt(0,nextpow2(numDataCarriers),0)  SampleTime=-1
  Constant1 : Constant  Value=true  SampleTime=-1
  Delay : Delay  DelayLength=1
  Delay1 : Delay  DelayLength=92  InitialCondition=0  UseCircularBuffer=on
  Delay2 : Delay  DelayLength=92
  Delay23 : Delay  DelayLength=1  InitialCondition=0
  Delay24 : Delay  DelayLength=1  InitialCondition=0
  Delay25 : Delay  DelayLength=1  InitialCondition=0
  Delay28 : Delay  DelayLength=1
  Delay{3..6} (4 alike) : Delay  DelayLength=1  InitialCondition=0  UseCircularBuffer=on
  HDL Counter : hdlsllib/Sources/HDL Counter  CountType=Count limited  CountInit=0  CountStep=1  CountMax=numDataCarriers-1  CountFromType=Initial value  CountFrom=0  CountResetPort=on  CountLoadPort=off  CountEnbPort=on  CountDirPort=off  CountHitOutputPort=off  CountDataType=Unsigned  CountWordLen=nextpow2(numDataCarriers)  CountFracLen=0  CountSampTime=1
  HDL Counter1 : hdlsllib/Sources/HDL Counter  CountType=Count limited  CountInit=0  CountStep=1  CountMax=numDataCarriers-1  CountFromType=Initial value  CountFrom=0  CountResetPort=on  CountLoadPort=off  CountEnbPort=on  CountDirPort=off  CountHitOutputPort=off  CountDataType=Unsigned  CountWordLen=nextpow2(numDataCarriers)  CountFracLen=0  CountSampTime=1
  OFDM Equalizer : whdlmod/OFDM Equalizer  EqualizationMethod=ZF  MaxLenChEstiPerSym=numDataCarriers  resetPort=on
  Switch : Switch  Criteria=u2 ~= 0  SaturateOnIntegerOverflow=off  InputSameDT=off
  rising_edge_detector : $bdroot/rising_edge_detector  SystemSampleTime=-1  VariantActivationTime=update diagram  AllowFlexibleInterface=on  Latency=0  AutoFrameSizeCalculation=off
  rising_edge_detector1 : $bdroot/rising_edge_detector  SystemSampleTime=-1  VariantActivationTime=update diagram  AllowFlexibleInterface=on  Latency=0  AutoFrameSizeCalculation=off
  data_out : Outport
  valid_out : Outport  Port=2
  channel_est_out : Outport  Port=3
  wires:
  reset/1 -> OFDM Equalizer/6
  Delay6/1 -> Delay/1
  Delay5/1 -> Channel Estimates Store RAM/1
  Delay4/1 -> HDL Counter1/2, Delay28/1
  Delay3/1 -> HDL Counter/2, Channel Estimates Store RAM/3
  Delay1/1 -> channel_est_out/1
  dont_use_equalizer/1 -> Switch/2
  OFDM Equalizer/1 -> Switch/3
  Delay2/1 -> Switch/1
  rising_edge_detector1/1 -> HDL Counter/1
  rising_edge_detector/1 -> HDL Counter1/1
  Delay25/1 -> OFDM Equalizer/3  "Valid"
  Constant1/1 -> OFDM Equalizer/5
  Constant/1 -> OFDM Equalizer/4
  Delay24/1 -> Delay2/1, OFDM Equalizer/1
  Channel Estimates Store RAM/1 -> Delay23/1
  HDL Counter1/1 -> Channel Estimates Store RAM/4  "rdAddr"
  valid_data/1 -> Delay4/1, rising_edge_detector/1
  valid_channel_estimate/1 -> Delay3/1, rising_edge_detector1/1
  HDL Counter/1 -> Channel Estimates Store RAM/2
  Delay/1 -> Delay24/1
  Delay28/1 -> Delay25/1
  OFDM Equalizer/2 -> valid_out/1
  data_in/1 -> Delay6/1
  Switch/1 -> data_out/1
  channel_estimate_in/1 -> Delay5/1
  Delay23/1 -> OFDM Equalizer/2, Delay1/1  "hEst"

== system HDL_ieee_8021513/channel_estimation_and_equalization/Channel Estimation ==
  note: Reference signal sub carriers are stored in LUT.
  data_in : Inport
  valid_in : Inport  Port=2
  reset : Inport  Port=3
  Constant : Constant  Value=numDataCarriers  OutDataTypeStr=fixdt(0,nextpow2(numDataCarriers),0)  SampleTime=-1
  Delay{1..4,7} (5 alike) : Delay  DelayLength=1  InitialCondition=0
  Direct Lookup Table (n-D) : LookupNDDirect  NumberOfTableDimensions=1  Table=fi(channelEstReference, 1, 16, 12)  DiagnosticForOutOfRangeInput=Error  RemoveProtectionInput=on  TableDataTypeStr=fixdt(1,16,12)
  HDL Counter : hdlsllib/Sources/HDL Counter  CountType=Count limited  CountInit=0  CountStep=1  CountMax=numDataCarriers-1  CountFromType=Initial value  CountFrom=0  CountResetPort=on  CountLoadPort=off  CountEnbPort=on  CountDirPort=off  CountHitOutputPort=off  CountDataType=Unsigned  CountWordLen=nextpow2(numDataCarriers)  CountFracLen=0  CountSampTime=1
  OFDM Channel Estimator : whdlmod/OFDM Channel Estimator  timeAvgCheckBox=on  numOFDMSymToBeAvg=2  enableInterpCheckBox=off  interpFac=3  maxNumSubCarPerSym=N  resetPort=on
  rising_edge_detector : $bdroot/rising_edge_detector  SystemSampleTime=-1  VariantActivationTime=update diagram  AllowFlexibleInterface=on  Latency=0  AutoFrameSizeCalculation=off
  channel_estimate : Outport
  valid_estimate : Outport  Port=2
  wires:
  reset/1 -> OFDM Channel Estimator/6
  rising_edge_detector/1 -> HDL Counter/1
  Delay2/1 -> Delay4/1
  Delay3/1 -> OFDM Channel Estimator/2, OFDM Channel Estimator/4
  Delay7/1 -> OFDM Channel Estimator/3
  Delay4/1 -> OFDM Channel Estimator/1
  HDL Counter/1 -> Direct Lookup Table (n-D)/1
  Delay1/1 -> Delay3/1, HDL Counter/2
  data_in/1 -> Delay2/1
  OFDM Channel Estimator/2 -> valid_estimate/1
  Direct Lookup Table (n-D)/1 -> Delay7/1
  valid_in/1 -> Delay1/1, rising_edge_detector/1
  Constant/1 -> OFDM Channel Estimator/5
  OFDM Channel Estimator/1 -> channel_estimate/1

== system HDL_ieee_8021513/constellation_descrambler/rotate_-90 ==
  data_in : Inport
  valid_in : Inport  Port=2
  s1_in : Inport  Port=3
  s2_in : Inport  Port=4
  Delay : Delay  InitialCondition=0  UseCircularBuffer=on
  Delay1 : Delay  InitialCondition=0  UseCircularBuffer=on
  Delay2 : Delay  DelayLength=1  InitialCondition=0  UseCircularBuffer=on
  Delay3 : Delay  DelayLength=1  InitialCondition=0  UseCircularBuffer=on
  rotate_-90 : Subsystem
  data_out : Outport  VectorParamsAs1DForOutWhenUnconnected=off
  valid_out : Outport  Port=2  VectorParamsAs1DForOutWhenUnconnected=off
  wires:
  s2_in/1 -> rotate_-90/1(s2)  "s2"
  s1_in/1 -> rotate_-90/2(s1)  "s1"
  Delay3/1 -> valid_out/1
  Delay2/1 -> data_out/1  "data_out"
  Delay1/1 -> Delay3/1
  rotate_-90/1(data_out) -> Delay2/1  "data_out"
  Delay/1 -> rotate_-90/3(data_in)  "data_in"
  data_in/1 -> Delay/1
  valid_in/1 -> Delay1/1  "en"

== system HDL_ieee_8021513/constellation_scrambler/rotate ==
  s2 : Inport
  s1 : Inport  Port=2
  data_in : Inport  Port=3
  Bit Concat : hdlsllib/Logic and Bit Operations/Bit Concat  numInputs=2
  Complex to Real-Imag : ComplexToRealImag
  Complex to Real-Imag1 : ComplexToRealImag
  Complex to Real-Imag2 : ComplexToRealImag
  Multiport Switch : MultiPortSwitch  DataPortOrder=Zero-based contiguous  Inputs=4  zeroidx=on  SaturateOnIntegerOverflow=off  InputSameDT=off
  Real-Imag to Complex : RealImagToComplex
  Real-Imag to Complex1 : RealImagToComplex
  Real-Imag to Complex2 : RealImagToComplex
  Unary Minus{,1..3} (4 alike) : UnaryMinus
  data_out : Outport
  wires:
  s2/1 -> Bit Concat/1
  s1/1 -> Bit Concat/2
  Bit Concat/1 -> Multiport Switch/1
  data_in/1 -> Complex to Real-Imag1/1, Complex to Real-Imag2/1, Complex to Real-Imag/1, Multiport Switch/2
  Complex to Real-Imag/1 -> Unary Minus/1
  Unary Minus/1 -> Real-Imag to Complex/1
  Complex to Real-Imag/2 -> Unary Minus3/1
  Real-Imag to Complex/1 -> Multiport Switch/4
  Complex to Real-Imag1/1 -> Real-Imag to Complex1/2
  Complex to Real-Imag1/2 -> Unary Minus1/1
  Unary Minus1/1 -> Real-Imag to Complex1/1
  Real-Imag to Complex1/1 -> Multiport Switch/3
  Complex to Real-Imag2/1 -> Unary Minus2/1
  Unary Minus2/1 -> Real-Imag to Complex2/2
  Complex to Real-Imag2/2 -> Real-Imag to Complex2/1
  Real-Imag to Complex2/1 -> Multiport Switch/5
  Multiport Switch/1 -> data_out/1
  Unary Minus3/1 -> Real-Imag to Complex/2

== system HDL_ieee_8021513/downshifter/digital_carrier_receiver ==
  dataIn : Inport
  ncoIn : Inport  Port=2
  Complex to Real-Imag : ComplexToRealImag
  Constant : Constant  Value=2  OutDataTypeStr=Inherit: Inherit via back propagation  SampleTime=-1
  Delay{,1..4} (5 alike) : Delay  InitialCondition=0  UseCircularBuffer=on
  Product : Product  OutDataTypeStr=Inherit: Same as first input
  Product1 : Product  InputSameDT=on  OutDataTypeStr=Inherit: Same as first input
  Product2 : Product  OutDataTypeStr=Inherit: Same as first input
  Real-Imag to Complex : RealImagToComplex
  Unary Minus : UnaryMinus
  data_out : Outport  VectorParamsAs1DForOutWhenUnconnected=off
  wires:
  Real-Imag to Complex/1 -> data_out/1
  Delay/1 -> Real-Imag to Complex/1
  Delay4/1 -> Real-Imag to Complex/2
  Product/1 -> Delay/1
  Product2/1 -> Delay4/1
  Complex to Real-Imag/2 -> Product2/2
  Delay3/1 -> Product2/1
  Complex to Real-Imag/1 -> Product/2
  Delay2/1 -> Complex to Real-Imag/1
  Unary Minus/1 -> Delay3/1
  Product1/1 -> Delay2/1
  Delay1/1 -> Product/1
  Constant/1 -> Product1/1
  ncoIn/1 -> Product1/2
  dataIn/1 -> Delay1/1, Unary Minus/1

== system HDL_ieee_8021513/frequency_upshift/Mixer ==
  dataIn : Inport
  ncoIn : Inport  Port=2
  Add : Sum  Inputs=+-  InputSameDT=on  OutDataTypeStr=Inherit: Same as first input
  Complex to Real-Imag : ComplexToRealImag
  Complex to Real-Imag1 : ComplexToRealImag
  Delay{1..4} (4 alike) : Delay  InitialCondition=0
  Delay12 : Delay  DelayLength=1  InitialCondition=0
  Delay6 : Delay  DelayLength=1  InitialCondition=0
  Delay7 : Delay  DelayLength=1  InitialCondition=0
  Product1 : Product  OutDataTypeStr=Inherit: Same as first input
  Product2 : Product  OutDataTypeStr=Inherit: Same as first input
  mixedOut : Outport
  wires:
  Delay1/1 -> Product1/1
  ncoIn/1 -> Complex to Real-Imag1/1
  Product1/1 -> Delay6/1
  Product2/1 -> Delay7/1
  Delay7/1 -> Add/2
  Complex to Real-Imag1/2 -> Delay4/1
  Complex to Real-Imag/1 -> Delay1/1
  Delay6/1 -> Add/1
  Add/1 -> Delay12/1
  Delay4/1 -> Product2/2
  Delay2/1 -> Product2/1
  Delay12/1 -> mixedOut/1
  dataIn/1 -> Complex to Real-Imag/1
  Complex to Real-Imag1/1 -> Delay3/1
  Delay3/1 -> Product1/2
  Complex to Real-Imag/2 -> Delay2/1

== system HDL_ieee_8021513/full_ofdm_modulator/enabled_qam_and_scrambler ==
  data_in : Inport
  valid_in : Inport  Port=2
  bits_per_subcarrier : Inport  Port=3
  init : Inport  Port=4
  new : Inport  Port=5
  cp_len : Inport  Port=6
  s2_in : Inport  Port=7
  s1_in : Inport  Port=8
  Enable : EnablePort
  Delay : Delay  DelayLength=1  InitialCondition=0  UseCircularBuffer=on
  Delay1 : Delay  DelayLength=1  InitialCondition=0  UseCircularBuffer=on
  Delay2 : Delay  DelayLength=1  InitialCondition=0  UseCircularBuffer=on
  Delay3 : Delay  DelayLength=3  InitialCondition=0  UseCircularBuffer=on
  constellation_scrambler : $bdroot/constellation_scrambler  SystemSampleTime=-1  VariantActivationTime=update diagram  AllowFlexibleInterface=on  Latency=0  AutoFrameSizeCalculation=off
  qam_mod : $bdroot/qam_mod  SystemSampleTime=-1  VariantActivationTime=update diagram  AllowFlexibleInterface=on  Latency=0  AutoFrameSizeCalculation=off
  data_out : Outport  VectorParamsAs1DForOutWhenUnconnected=off
  valid_out : Outport  Port=2  VectorParamsAs1DForOutWhenUnconnected=off
  cp_len_out : Outport  Port=3  VectorParamsAs1DForOutWhenUnconnected=off
  valid_scrambler : Outport  Port=4  VectorParamsAs1DForOutWhenUnconnected=off
  init_out : Outport  Port=5  VectorParamsAs1DForOutWhenUnconnected=off
  new_out : Outport  Port=6  VectorParamsAs1DForOutWhenUnconnected=off
  wires:
  Delay2/1 -> Delay3/1
  cp_len/1 -> Delay2/1
  Delay3/1 -> cp_len_out/1
  new/1 -> Delay1/1
  Delay1/1 -> new_out/1
  init/1 -> Delay/1
  Delay/1 -> init_out/1
  s1_in/1 -> constellation_scrambler/3
  s2_in/1 -> constellation_scrambler/4
  qam_mod/2 -> constellation_scrambler/2, valid_scrambler/1
  qam_mod/1 -> constellation_scrambler/1
  constellation_scrambler/2 -> valid_out/1
  constellation_scrambler/1 -> data_out/1  "out_new"
  bits_per_subcarrier/1 -> qam_mod/3
  data_in/1 -> qam_mod/1
  valid_in/1 -> qam_mod/2

== system HDL_ieee_8021513/full_rx/cpid_to_cplen ==
  cp_id : Inport
  Bits to Word : hdlsllib/Logic and Bit Operations/Bits to Word
  Constant3 : Constant  Value=N/32  OutDataTypeStr=fixdt(0,4,0)  SampleTime=-1
  Data Type Conversion : DataTypeConversion  OutDataTypeStr=fixdt(0,1,0)  SaturateOnIntegerOverflow=off  RndMeth=Floor
  Delay1 : Delay  DelayLength=1  InitialCondition=0  UseCircularBuffer=on
  Product : Product  OutDataTypeStr=uint8
  payload_cp_len : Outport
  wires:
  cp_id/1 -> Data Type Conversion/1
  Data Type Conversion/1 -> Bits to Word/1
  Product/1 -> Delay1/1
  Bits to Word/1 -> Product/2
  Constant3/1 -> Product/1
  Delay1/1 -> payload_cp_len/1
